simulink model "Project1_Part2"  (R2023b)
settings: Solver=VariableStepAuto  StartTime=0.0  StopTime=10.0  RelTol=1e-3
values from neighbouring files (symbols this model uses):
  A = T_0_values(l)    [Project1_Part2.m]    (also in Project1_Part2_Option1_CODE.m = A_values(j); Project1_Part2_Option2_CODE.m = A_values(j); Project1_Part2_Option3_CODE.m = A_values(j))
  J2 = 1    [Project1_Part2.m]    (also in Project1_Part2_Option1_CODE.m; Project1_Part2_Option2_CODE.m; Project1_Part2_Option3_CODE.m)
  k = k_values(i)    [Project1_Part2.m]    (also in Project1_Part2_Option1_CODE.m)
  w_0 = 5    [Project1_Part2.m]
undefined symbols (not defined in the file or in its folder): b, J
settings Model: Creator=turtl  LastModifiedBy=turtl

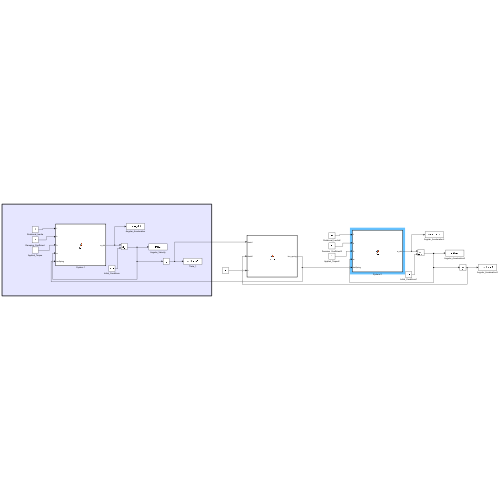
[thumbnail: Simulink's stored preview of the top-level diagram]
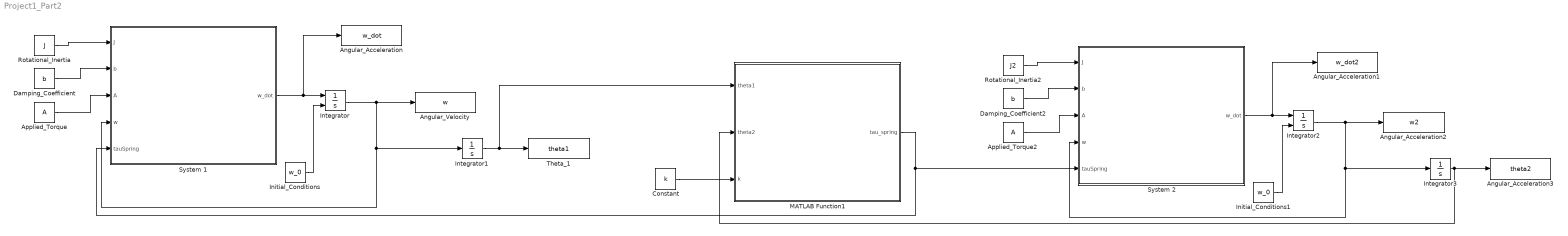
== system Project1_Part2 ==
  Angular_Acceleration : ToWorkspace  VariableName=w_dot  SaveFormat=Timeseries  SampleTime=-1
  Angular_Acceleration1 : ToWorkspace  VariableName=w_dot2  SaveFormat=Timeseries  SampleTime=-1
  Angular_Acceleration2 : ToWorkspace  VariableName=w2  SaveFormat=Timeseries  SampleTime=-1
  Angular_Acceleration3 : ToWorkspace  VariableName=theta2  SaveFormat=Timeseries  SampleTime=-1
  Angular_Velocity : ToWorkspace  VariableName=w  SaveFormat=Timeseries  SampleTime=-1
  Applied_Torque : Constant  Value=A
  Applied_Torque2 : Constant  Value=A
  Constant : Constant  Value=k
  Damping_Coefficient : Constant  Value=b
  Damping_Coefficient2 : Constant  Value=b
  Initial_Conditions : Constant  Value=w_0
  Initial_Conditions1 : Constant  Value=w_0
  Integrator : Integrator  InitialConditionSource=external  LimitOutput=on  UpperSaturationLimit=10000  LowerSaturationLimit=0
  Integrator1 : Integrator
  Integrator2 : Integrator  InitialConditionSource=external  LimitOutput=on  UpperSaturationLimit=10000  LowerSaturationLimit=0
  Integrator3 : Integrator
  MATLAB Function1 : MATLAB Function  TreatAsAtomicUnit=on
  Rotational_Inertia : Constant  Value=J
  Rotational_Inertia2 : Constant  Value=J2
  System 1 : MATLAB Function  TreatAsAtomicUnit=on
  System 2 : MATLAB Function  TreatAsAtomicUnit=on
  Theta_1 : ToWorkspace  VariableName=theta1  SaveFormat=Timeseries  SampleTime=-1
  wires:
  Applied_Torque/1 -> System 1/3(A)
  Integrator2/1 -> Angular_Acceleration2/1, Integrator3/1, System 2/4(w)
  Initial_Conditions1/1 -> Integrator2/2
  Rotational_Inertia2/1 -> System 2/1(J)
  Applied_Torque2/1 -> System 2/3(A)
  Rotational_Inertia/1 -> System 1/1(J)
  Integrator1/1 -> MATLAB Function1/1(theta1), Theta_1/1
  Damping_Coefficient2/1 -> System 2/2(b)
  System 1/1(w_dot) -> Angular_Acceleration/1, Integrator/1
  System 2/1(w_dot) -> Angular_Acceleration1/1, Integrator2/1
  Integrator/1 -> Angular_Velocity/1, Integrator1/1, System 1/4(w)
  Initial_Conditions/1 -> Integrator/2
  Damping_Coefficient/1 -> System 1/2(b)
  Constant/1 -> MATLAB Function1/3(k)
  Integrator3/1 -> MATLAB Function1/2(theta2), Angular_Acceleration3/1
  MATLAB Function1/1(tau_spring) -> System 2/5(tauSpring), System 1/5(tauSpring)

== matlab function Project1_Part2/MATLAB Function1 ==
  data: theta1 input; tau_spring output; theta2 input; k input
function tau_spring = spring(theta1,theta2,k)
tau_spring = k*(theta1-theta2);
end

== matlab function Project1_Part2/System 1 ==
  data: J input; w_dot output; b input; A input; w input; tauSpring input
function w_dot = fcn(J, b, A,w,tauSpring)
w_dot = (1/J)*(A-b*w-tauSpring);
end

== matlab function Project1_Part2/System 2 ==
  data: J input; w_dot output; b input; A input; w input; tauSpring input
function w_dot = fcn(J, b, A,w,tauSpring)
w_dot = (1/J)*(A-b*w+tauSpring);
end
